simulink model "SecondOrder_Sim"  (R2022b)
settings: Solver=VariableStepAuto  StartTime=0.0  StopTime=10.0  RelTol=1e-3
settings Model: Creator=MAAM  LastModifiedBy=MAAM

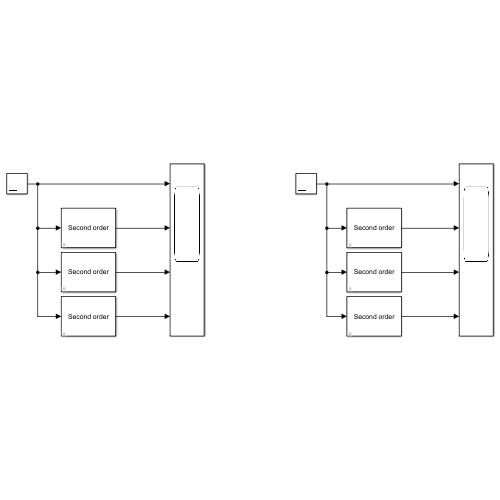
[thumbnail: Simulink's stored preview of the top-level diagram]
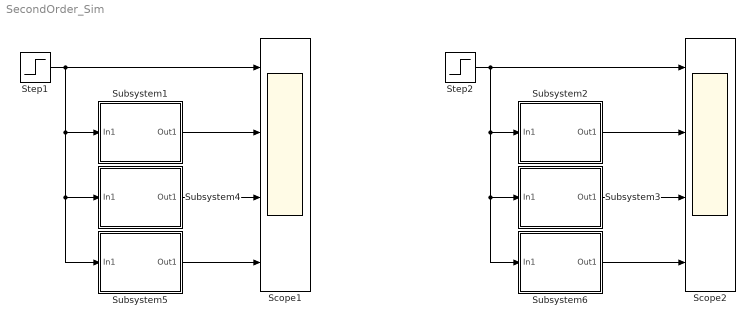
== system SecondOrder_Sim ==
  Scope1 : Scope  NumInputPorts=4
  Scope2 : Scope  NumInputPorts=4
  Step1 : Step  SampleTime=0
  Step2 : Step  SampleTime=0
  Subsystem1 : Subsystem  mask{W_n=1, Z=1}
      mask prompts: W_n "Natural frequency "\omega_n""; Z "Damping Constant "\zeta""
      mask Display: fprintf("Second order");
  Subsystem2 : Subsystem  mask{W_n=1, Z=0.5}
      mask prompts: W_n "Natural frequency "\omega_n""; Z "Damping Constant "\zeta""
      mask Display: fprintf("Second order");
  Subsystem3 : Subsystem  mask{W_n=1, Z=1}
      mask prompts: W_n "Natural frequency "\omega_n""; Z "Damping Constant "\zeta""
      mask Display: fprintf("Second order");
  Subsystem4 : Subsystem  mask{W_n=2, Z=1}
      mask prompts: W_n "Natural frequency "\omega_n""; Z "Damping Constant "\zeta""
      mask Display: fprintf("Second order");
  Subsystem5 : Subsystem  mask{W_n=3, Z=1}
      mask prompts: W_n "Natural frequency "\omega_n""; Z "Damping Constant "\zeta""
      mask Display: fprintf("Second order");
  Subsystem6 : Subsystem  mask{W_n=1, Z=1.5}
      mask prompts: W_n "Natural frequency "\omega_n""; Z "Damping Constant "\zeta""
      mask Display: fprintf("Second order");
  wires:
  Step1/1 -> Scope1/1, Subsystem1/1(In1), Subsystem5/1(In1), Subsystem4/1(In1)
  Step2/1 -> Subsystem2/1(In1), Subsystem3/1(In1), Subsystem6/1(In1), Scope2/1
  Subsystem2/1(Out1) -> Scope2/2
  Subsystem3/1(Out1) -> Scope2/3
  Subsystem6/1(Out1) -> Scope2/4
  Subsystem1/1(Out1) -> Scope1/2
  Subsystem4/1(Out1) -> Scope1/3
  Subsystem5/1(Out1) -> Scope1/4

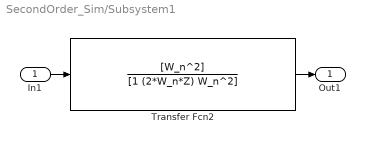
== system SecondOrder_Sim/Subsystem1 ==
  In1 : Inport
  Transfer Fcn2 : TransferFcn  Numerator=[W_n^2]  Denominator=[1 (2*W_n*Z) W_n^2]
  Out1 : Outport
  wires:
  In1/1 -> Transfer Fcn2/1
  Transfer Fcn2/1 -> Out1/1

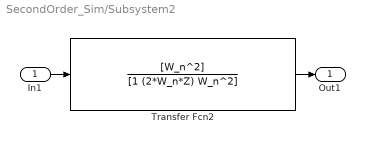
== system SecondOrder_Sim/Subsystem2 ==
  In1 : Inport
  Transfer Fcn2 : TransferFcn  Numerator=[W_n^2]  Denominator=[1 (2*W_n*Z) W_n^2]
  Out1 : Outport
  wires:
  Transfer Fcn2/1 -> Out1/1
  In1/1 -> Transfer Fcn2/1

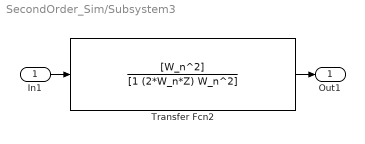
== system SecondOrder_Sim/Subsystem3 ==
  In1 : Inport
  Transfer Fcn2 : TransferFcn  Numerator=[W_n^2]  Denominator=[1 (2*W_n*Z) W_n^2]
  Out1 : Outport
  wires:
  In1/1 -> Transfer Fcn2/1
  Transfer Fcn2/1 -> Out1/1

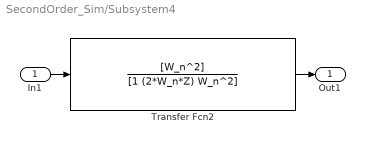
== system SecondOrder_Sim/Subsystem4 ==
  In1 : Inport
  Transfer Fcn2 : TransferFcn  Numerator=[W_n^2]  Denominator=[1 (2*W_n*Z) W_n^2]
  Out1 : Outport
  wires:
  Transfer Fcn2/1 -> Out1/1
  In1/1 -> Transfer Fcn2/1

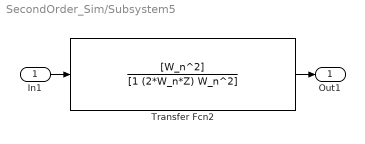
== system SecondOrder_Sim/Subsystem5 ==
  In1 : Inport
  Transfer Fcn2 : TransferFcn  Numerator=[W_n^2]  Denominator=[1 (2*W_n*Z) W_n^2]
  Out1 : Outport
  wires:
  In1/1 -> Transfer Fcn2/1
  Transfer Fcn2/1 -> Out1/1

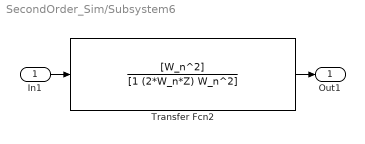
== system SecondOrder_Sim/Subsystem6 ==
  In1 : Inport
  Transfer Fcn2 : TransferFcn  Numerator=[W_n^2]  Denominator=[1 (2*W_n*Z) W_n^2]
  Out1 : Outport
  wires:
  Transfer Fcn2/1 -> Out1/1
  In1/1 -> Transfer Fcn2/1
